simulink model "Ejercicio_1"  (R2013a)
settings: Solver=ode45  StartTime=0.0  StopTime=10.0  RelTol=1e-3
libraries: simulink x1
settings Model: Creator=Miguel  LastModifiedBy=Miguel

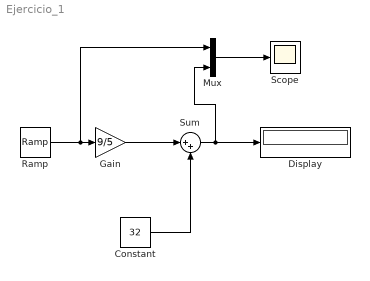
== system Ejercicio_1 ==
  Constant : Constant  Value=32
  Display : Display
  Gain : Gain  Gain=9/5
  Mux : Mux  Inputs=2
  Ramp : simulink/Sources/Ramp  slope=1  start=0  X0=0
  Scope : Scope
  Sum : Sum  Inputs=|++
  wires:
  Ramp/1 -> Mux/1, Gain/1
  Gain/1 -> Sum/1
  Constant/1 -> Sum/2
  Sum/1 -> Mux/2, Display/1
  Mux/1 -> Scope/1
